simulink model "Filter_design"  (R2020b)
settings: Solver=FixedStepDiscrete  StartTime=0.0  StopTime=0.5  FixedStep=1e-3  RelTol=1e-3
settings Model: Creator=luca9  LastModifiedBy=luca9
settings OptimizationCC: DefaultParameterBehavior=Inlined  EnhancedBackFolding=on  PassReuseOutputArgsAs=Individual arguments  ZeroExternalMemoryAtStartup=off  ZeroInternalMemoryAtStartup=off  OptimizeBlockOrder=speed  DifferentSizesBufferReuse=on  OptimizationCustomize=off  EfficientTunableParamExpr=on
settings DebuggingCC: ParameterTunabilityLossMsg=error
settings SFSimCC: MATLABDynamicMemAlloc=off
settings RTWCC: Description=Embedded Coder  SystemTargetFile=ert.tlc  TemplateMakefile=ert_default_tmf
settings CodeAppCC: ForceParamTrailComments=on  IgnoreCustomStorageClasses=off  OperatorAnnotations=on  SimulinkDataObjDesc=on  SFDataObjDesc=on  InsertBlockDesc=on
settings ERTTargetCC: TargetLangStandard=C99 (ISO)  GenerateSampleERTMain=on  InlinedParameterPlacement=NonHierarchical  ERTCustomFileTemplate=example_file_process.tlc

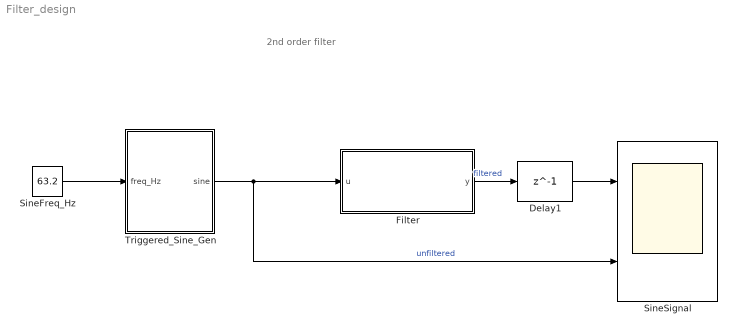
== system Filter_design ==
  note: 2nd order filter
  Delay1 : Delay  DelayLength=1  InitialCondition=0  UseCircularBuffer=on
  Filter : Subsystem
  SineFreq_Hz : Constant  Value=63.2
  SineSignal : Scope  NumInputPorts=2
  Triggered_Sine_Gen : Subsystem
  wires:
  Triggered_Sine_Gen/1(sine) -> SineSignal/2, Filter/1(u)  "unfiltered"
  Filter/1(y) -> Delay1/1  "filtered"
  SineFreq_Hz/1 -> Triggered_Sine_Gen/1(freq_Hz)
  Delay1/1 -> SineSignal/1

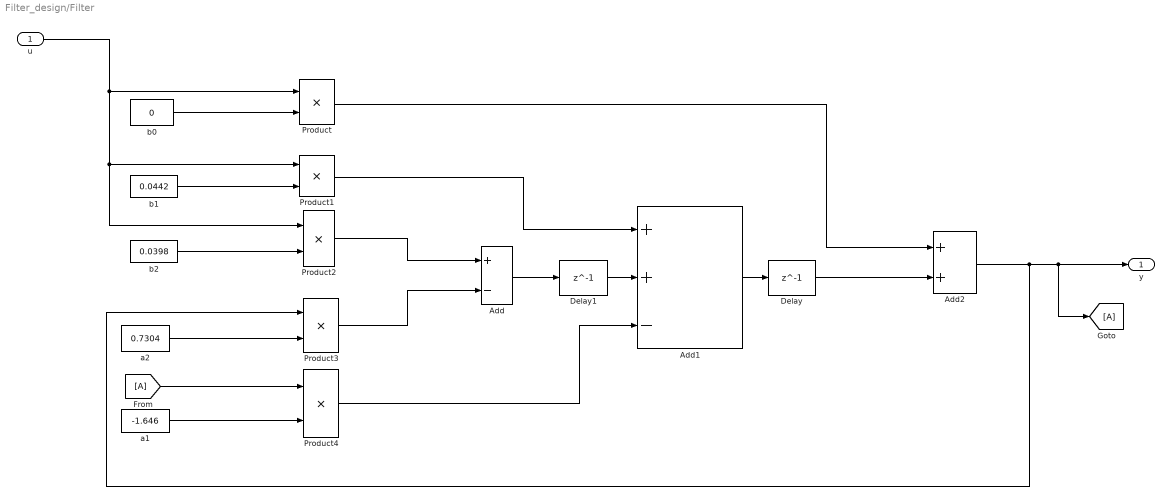
== system Filter_design/Filter ==
  u : Inport
  Add : Sum  Inputs=+-
  Add1 : Sum  Inputs=++-
  Add2 : Sum
  Delay : Delay  DelayLength=1  InitialCondition=0  UseCircularBuffer=on
  Delay1 : Delay  DelayLength=1  InitialCondition=0  UseCircularBuffer=on
  Product{,1..4} (5 alike) : Product
  a1 : Constant  Value=-1.646
  a2 : Constant  Value=0.7304
  b0 : Constant  Value=0
  b1 : Constant  Value=0.0442
  b2 : Constant  Value=0.0398
  y : Outport
  wires:
  Delay1/1 -> Add1/2
  Product3/1 -> Add/2
  Delay/1 -> Add2/2
  [A] -> Product4/1
  Product/1 -> Add2/1
  Add1/1 -> Delay/1
  Product1/1 -> Add1/1
  Add2/1 -> Product3/1, y/1, [A]
  b0/1 -> Product/2
  b2/1 -> Product2/2
  u/1 -> Product/1, Product1/1, Product2/1
  Product4/1 -> Add1/3
  b1/1 -> Product1/2
  Product2/1 -> Add/1
  Add/1 -> Delay1/1
  a2/1 -> Product3/2
  a1/1 -> Product4/2

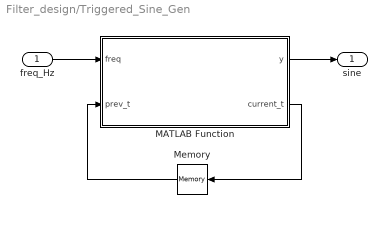
== system Filter_design/Triggered_Sine_Gen ==
  freq_Hz : Inport
  MATLAB Function : MATLAB Function  TreatAsAtomicUnit=on
  Memory : Memory  InheritSampleTime=on
  sine : Outport
  wires:
  Memory/1 -> MATLAB Function/2(prev_t)
  MATLAB Function/1(y) -> sine/1
  MATLAB Function/2(current_t) -> Memory/1
  freq_Hz/1 -> MATLAB Function/1(freq)

== matlab function Filter_design/Triggered_Sine_Gen/MATLAB Function ==
  data: freq input; y output; prev_t input; current_t output
function [y, current_t] = fcn(freq, prev_t)

y = sin(prev_t*0.001*pi*2*freq)
if(prev_t < 1e6)
    current_t=prev_t+1;
else
    current_t=0;
end
